simulink model "EnabledSubSystem"  (Simulink 7.4)
settings: Solver=VariableStepDiscrete  StartTime=0.0  StopTime=10.0  MaxStep=1  RelTol=1e-3
settings Model: Creator=dread  LastModifiedBy=dread

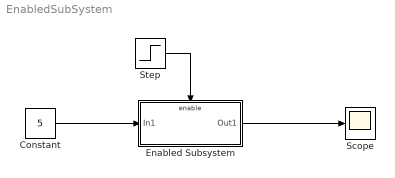
== system EnabledSubSystem ==
  Constant : Constant  Value=5  OutDataType=fixdt(1, 16)  OutScaling=2^0
  Enabled Subsystem : Subsystem  TreatAsAtomicUnit=on
  Scope : Scope
  Step : Step  Time=5  SampleTime=0
  wires:
  Constant/1 -> Enabled Subsystem/1(In1)
  Enabled Subsystem/1(Out1) -> Scope/1
  Step/1 -> Enabled Subsystem/Enable

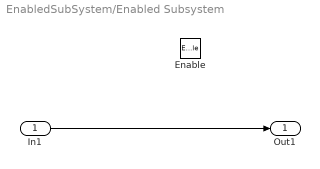
== system EnabledSubSystem/Enabled Subsystem ==
  In1 : Inport  OutDataType=fixdt(1, 16)  OutScaling=2^0
  Enable : EnablePort
  Out1 : Outport  OutDataType=fixdt(1, 16)  OutScaling=2^0
  wires:
  In1/1 -> Out1/1
